simulink model "attitude_controller"  (R2024b)
settings: Solver=ode1  StartTime=0.0  StopTime=120  FixedStep=0.1  RelTol=1e-3
values from neighbouring files (symbols this model uses):
  g0 = 9.81    [main.m]
  m_0 = 6492 * 1000    (= 6492000)    [main.m]
  m_dot_e = T_e_with_losses/v_ex    (= 799.471894568)    [main.m]
  m_p_0 = 4165 * 1000    (= 4165000)    [main.m]
  n_eg_g = 3 + 12    (= 15)    [main.m]
  n_eg_ng = 26    [main.m]
  T_g_full_throttle = T_e_with_losses * n_eg_g    (= 41174801.25)    [main.m]
  T_ng_full_throttle = T_e_with_losses * n_eg_ng    (= 71369655.5)    [main.m]
  theta_0 = deg2rad(90)    [main.m]
  theta_ref = a0 + a1 * t + a2 * t.^2 + a3 * t.^3    [main.m]
libraries: simulink_extras x3, slpidlib x1
settings Model: Creator=jonathanvanzyl  LastModifiedBy=jonathanvanzyl

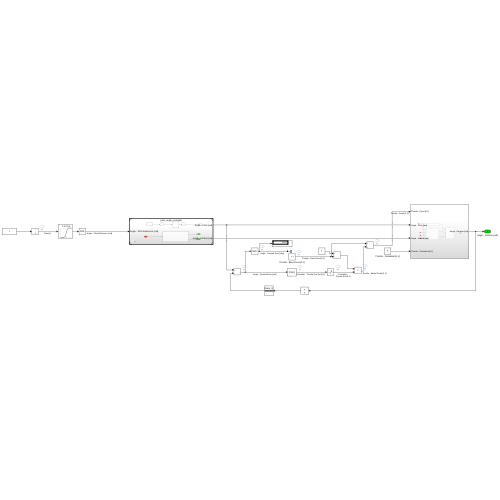
[thumbnail: Simulink's stored preview of the top-level diagram]
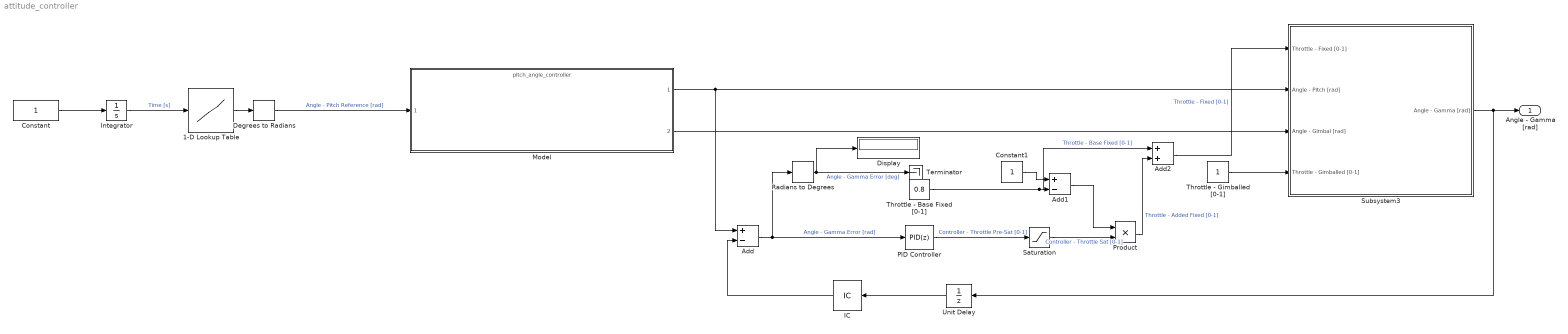
== system attitude_controller ==
  1-D Lookup Table : Lookup_n-D  NumberOfTableDimensions=1  BreakpointsForDimension1=t  Table=theta_ref  InternalRulePriority=Speed  RndMeth=Simplest
  Add : Sum  Inputs=+-
  Add1 : Sum  Inputs=+-
  Add2 : Sum
  Constant : Constant
  Constant1 : Constant
  Degrees to Radians : simulink_extras/Transformations/Degrees to Radians
  Display : Display
  IC : InitialCondition  Value=theta_0
  Integrator : Integrator
  Model : ModelReference  ModelNameDialog=pitch_angle_controller  SimulationMode=Normal  ModelReferenceVersion=1.17
  PID Controller : slpidlib/PID Controller  Controller=PID  Form=Parallel  TimeDomain=Discrete-time  UseExternalTs=off  SampleTime=-1  IntegratorMethod=Forward Euler  FilterMethod=Forward Euler  ControllerParametersSource=internal  P=100  I=0  UseKiTs=off  D=0  UseExternalDerivativeSource=off  N=0.0005  UseFilter=on  TunerSelectOption=Transfer Function Based (PID Tuner App)  InitialConditionSource=internal  InitialConditionForIntegrator=0  InitialConditionForFilter=0  DifferentiatorICPrevScaledInput=0  ExternalReset=none  TrackingMode=off  Kt=1  LimitOutput=off  SatLimitsSource=internal  UpperSaturationLimit=inf  LowerSaturationLimit=-inf  LinearizeAsGain=on  AntiWindupMode=none  Kb=1  LimitIntegrator=off  UpperIntegratorSaturationLimit=inf  LowerIntegratorSaturationLimit=-inf  POutMin=[]  POutMax=[]  IOutMin=[]  IOutMax=[]  DOutMin=[]  DOutMax=[]  NOutMin=[]  NOutMax=[]  SumOutMin=[]  SumOutMax=[]  SaturationOutMin=[]  SaturationOutMax=[]  PParamMin=[]  PParamMax=[]  IParamMin=[]  IParamMax=[]  DParamMin=[]  DParamMax=[]  NParamMin=[]  NParamMax=[]  KbParamMin=[]  KbParamMax=[]  KtParamMin=[]  KtParamMax=[]  KbOutMin=[]  KbOutMax=[]  KtOutMin=[]  KtOutMax=[]  IntegratorOutMin=[]  IntegratorOutMax=[]  FilterOutMin=[]  FilterOutMax=[]  SumI1OutMin=[]  SumI1OutMax=[]  SumI2OutMin=[]  SumI2OutMax=[]  SumI3OutMin=[]  SumI3OutMax=[]  SumI4OutMin=[]  SumI4OutMax=[]  SumDOutMin=[]  SumDOutMax=[]  DifferentiatorOutMin=[]  DifferentiatorOutMax=[]  FilterDiffOutCoefMin=[]  FilterDiffOutCoefMax=[]  ReciprocalOutMin=[]  ReciprocalOutMax=[]  SumDenOutMin=[]  SumDenOutMax=[]  SumNumOutMin=[]  SumNumOutMax=[]  DivideOutMin=[]  DivideOutMax=[]  UdiffTsProdOutMin=[]  UdiffTsProdOutMax=[]  NTsProdOutMin=[]  NTsProdOutMax=[]  UintegralTsProdOutMin=[]  UintegralTsProdOutMax=[]  UngainTsProdOutMin=[]  UngainTsProdOutMax=[]  ClampingZeroOutDataTypeStr=Inherit: Inherit via back propagation  ClampingZeroOutMin=[]  ClampingZeroOutMax=[]  FilterDenConstantOutDataTypeStr=Inherit: Inherit via back propagation  FilterDenConstantOutMin=[]  FilterDenConstantOutMax=[]  PCopyOutDataTypeStr=Inherit: Inherit via back propagation  PCopyOutMin=[]  PCopyOutMax=[]  NCopyOutDataTypeStr=Inherit: Inherit via back propagation  NCopyOutMin=[]  NCopyOutMax=[]  IntegratorContinuousStateAttributes=''  IntegratorStateMustResolveToSignalObject=off  IntegratorRTWStateStorageClass=Auto  FilterContinuousStateAttributes=''  FilterStateMustResolveToSignalObject=off  FilterRTWStateStorageClass=Auto  ParallelPVariant=InternalParameters  IdealPVariant=Disabled  IVariant=InternalParameters  DVariant=InternalParameters  IntegratorVariant=Discrete  SatVariant=Disabled  AWVariant=Passthrough  PCopyVariant=Disabled  TRVariant=Disabled  FdbkBlocksVariant=Forward  IdealPFdbkVariant=Disabled  SatFdbkVariant=Disabled  DerivativeFilterVariant=ForwardEulerFilter  NVariant=InternalParameters  NCopyVariant=Disabled  FilterICVariant=InternalICsFilter  IntegratorICVariant=InternalICs  ExternalResetVariant=Disabled  TRSumVariant=Passthrough  SumFdbkVariant=Disabled  SumVariant=Sum_PID  TsampFilterVariant=InternalTs  TsampNgainVariant=Passthrough  TsampIntegralVariant=Disabled_SignalSpec  ExternalSaturationOutDataTypeStr=Inherit: Same as second input  DerivativeSourceVariant=ErrorSignal  PreIntVariant=InternalPreInt
  Product : Product
  Radians to Degrees : simulink_extras/Transformations/Radians to Degrees
  Saturation : Saturate  UpperLimit=1  LowerLimit=0
  Subsystem3 : Subsystem
  Terminator : Terminator
  Throttle - Base Fixed [0-1] : Constant  Value=0.8
  Throttle - Gimballed [0-1] : Constant
  Unit Delay : UnitDelay  SampleTime=-1  HasFrameUpgradeWarning=on
  Angle - Gamma [rad] : Outport
  wires:
  Model/1 -> Add/1, Subsystem3/2(Angle - Pitch [rad])
  Model/2 -> Subsystem3/3(Angle - Gimbal [rad])
  Throttle - Gimballed [0-1]/1 -> Subsystem3/4(Throttle - Gimballed [0-1])
  Subsystem3/1(Angle - Gamma [rad]) -> Unit Delay/1, Angle - Gamma [rad]/1
  Unit Delay/1 -> IC/1
  IC/1 -> Add/2
  Add/1 -> Radians to Degrees/1, PID Controller/1  "Angle - Gamma Error [rad]"
  Add2/1 -> Subsystem3/1(Throttle - Fixed [0-1])  "Throttle - Fixed [0-1]"
  Constant/1 -> Integrator/1
  Integrator/1 -> 1-D Lookup Table/1  "Time [s]"
  1-D Lookup Table/1 -> Degrees to Radians/1
  Degrees to Radians/1 -> Model/1  "Angle - Pitch Reference [rad]"
  Radians to Degrees/1 -> Display/1, Terminator/1  "Angle - Gamma Error [deg]"
  PID Controller/1 -> Saturation/1  "Controller - Throttle Pre-Sat [0-1]"
  Add1/1 -> Product/1
  Throttle - Base Fixed [0-1]/1 -> Add2/1, Add1/2  "Throttle - Base Fixed [0-1]"
  Constant1/1 -> Add1/1
  Saturation/1 -> Product/2  "Controller - Throttle Sat [0-1]"
  Product/1 -> Add2/2  "Throttle - Added Fixed [0-1]"

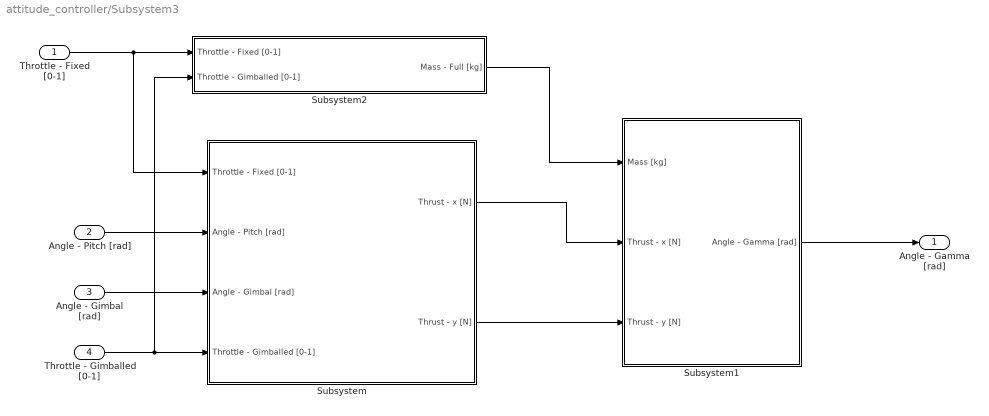
== system attitude_controller/Subsystem3 ==
  Throttle - Fixed [0-1] : Inport
  Angle - Pitch [rad] : Inport  Port=2
  Angle - Gimbal [rad] : Inport  Port=3
  Throttle - Gimballed [0-1] : Inport  Port=4
  Subsystem : Subsystem
  Subsystem1 : Subsystem
  Subsystem2 : Subsystem
  Angle - Gamma [rad] : Outport
  wires:
  Angle - Gimbal [rad]/1 -> Subsystem/3(Angle - Gimbal [rad])
  Subsystem2/1(Mass - Full [kg]) -> Subsystem1/1(Mass [kg])
  Subsystem/1(Thrust - x [N]) -> Subsystem1/2(Thrust - x [N])
  Subsystem/2(Thrust - y [N]) -> Subsystem1/3(Thrust - y [N])
  Angle - Pitch [rad]/1 -> Subsystem/2(Angle - Pitch [rad])
  Throttle - Fixed [0-1]/1 -> Subsystem/1(Throttle - Fixed [0-1]), Subsystem2/1(Throttle - Fixed [0-1])
  Subsystem1/1(Angle - Gamma [rad]) -> Angle - Gamma [rad]/1
  Throttle - Gimballed [0-1]/1 -> Subsystem2/2(Throttle - Gimballed [0-1]), Subsystem/4(Throttle - Gimballed [0-1])

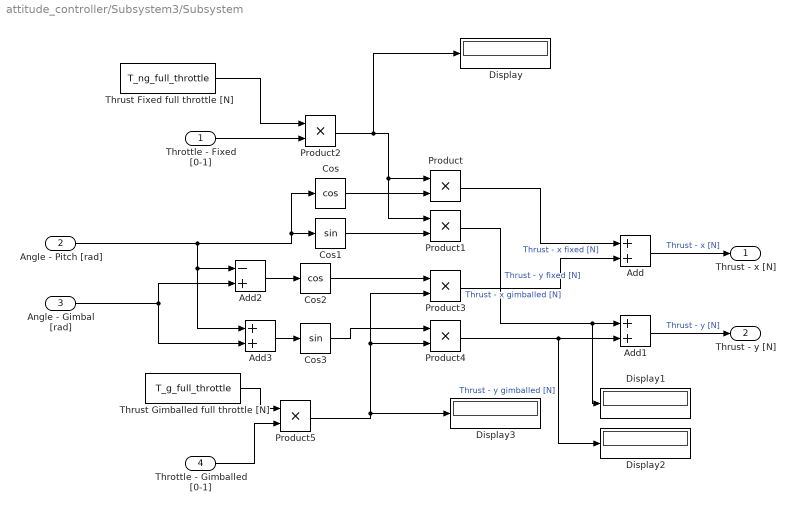
== system attitude_controller/Subsystem3/Subsystem ==
  Throttle - Fixed [0-1] : Inport
  Angle - Pitch [rad] : Inport  Port=2
  Angle - Gimbal [rad] : Inport  Port=3
  Throttle - Gimballed [0-1] : Inport  Port=4
  Add : Sum
  Add1 : Sum
  Add2 : Sum  Inputs=-+
  Add3 : Sum
  Cos : Trigonometry  Operator=cos
  Cos1 : Trigonometry
  Cos2 : Trigonometry  Operator=cos
  Cos3 : Trigonometry
  Display{,1..3} (4 alike) : Display
  Product{,1..5} (6 alike) : Product
  Thrust Fixed full throttle [N] : Constant  Value=T_ng_full_throttle
  Thrust Gimballed full throttle [N] : Constant  Value=T_g_full_throttle
  Thrust - x [N] : Outport
  Thrust - y [N] : Outport  Port=2
  wires:
  Add/1 -> Thrust - x [N]/1  "Thrust - x [N]"
  Thrust Gimballed full throttle [N]/1 -> Product5/1
  Product3/1 -> Add/2  "Thrust - x gimballed [N]"
  Product4/1 -> Display2/1, Add1/2  "Thrust - y gimballed [N]"
  Product5/1 -> Product3/2, Product4/2, Display3/1
  Cos2/1 -> Product3/1
  Angle - Gimbal [rad]/1 -> Add2/2, Add3/2
  Add3/1 -> Cos3/1
  Product/1 -> Add/1  "Thrust - x fixed [N]"
  Throttle - Fixed [0-1]/1 -> Product2/2
  Throttle - Gimballed [0-1]/1 -> Product5/2
  Thrust Fixed full throttle [N]/1 -> Product2/1
  Add2/1 -> Cos2/1
  Cos3/1 -> Product4/1
  Cos/1 -> Product/2
  Angle - Pitch [rad]/1 -> Add3/1, Add2/1, Cos/1, Cos1/1
  Add1/1 -> Thrust - y [N]/1  "Thrust - y [N]"
  Product1/1 -> Display1/1, Add1/1  "Thrust - y fixed [N]"
  Cos1/1 -> Product1/2
  Product2/1 -> Display/1, Product1/1, Product/1

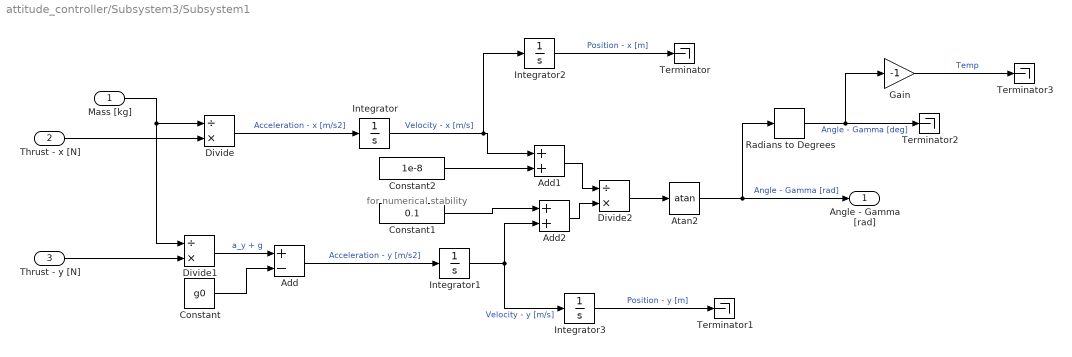
== system attitude_controller/Subsystem3/Subsystem1 ==
  note: for numerical stability
  Mass [kg] : Inport
  Thrust - x [N] : Inport  Port=2
  Thrust - y [N] : Inport  Port=3
  Add : Sum  Inputs=+-
  Add1 : Sum
  Add2 : Sum
  Atan2 : Trigonometry  Operator=atan
  Constant : Constant  Value=g0
  Constant1 : Constant  Value=0.1
  Constant2 : Constant  Value=1e-8
  Divide : Product  Inputs=/*
  Divide1 : Product  Inputs=/*
  Divide2 : Product  Inputs=/*
  Gain : Gain  Gain=-1
  Integrator{,1..3} (4 alike) : Integrator
  Radians to Degrees : simulink_extras/Transformations/Radians to Degrees
  Terminator{,1..3} (4 alike) : Terminator
  Angle - Gamma [rad] : Outport
  wires:
  Divide/1 -> Integrator/1  "Acceleration - x [m/s2]"
  Integrator2/1 -> Terminator/1  "Position - x [m]"
  Add/1 -> Integrator1/1  "Acceleration - y [m/s2]"
  Thrust - x [N]/1 -> Divide/2
  Constant1/1 -> Add2/1
  Integrator/1 -> Integrator2/1, Add1/1  "Velocity - x [m/s]"
  Add2/1 -> Divide2/2
  Integrator1/1 -> Integrator3/1, Add2/2  "Velocity - y [m/s]"
  Atan2/1 -> Radians to Degrees/1, Angle - Gamma [rad]/1  "Angle - Gamma [rad]"
  Thrust - y [N]/1 -> Divide1/2
  Divide1/1 -> Add/1  "a_y + g"
  Divide2/1 -> Atan2/1
  Constant2/1 -> Add1/2
  Add1/1 -> Divide2/1
  Constant/1 -> Add/2
  Integrator3/1 -> Terminator1/1  "Position - y [m]"
  Mass [kg]/1 -> Divide1/1, Divide/1
  Radians to Degrees/1 -> Gain/1, Terminator2/1  "Angle - Gamma [deg]"
  Gain/1 -> Terminator3/1  "Temp"

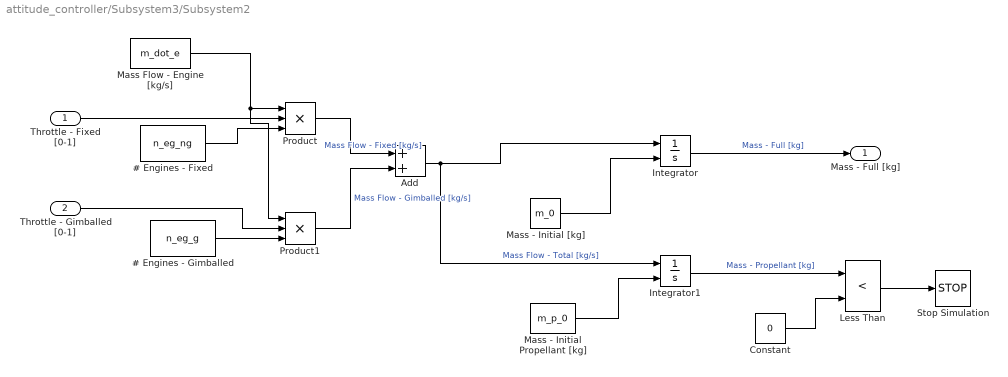
== system attitude_controller/Subsystem3/Subsystem2 ==
  Throttle - Fixed [0-1] : Inport
  Throttle - Gimballed [0-1] : Inport  Port=2
  # Engines - Fixed : Constant  Value=n_eg_ng
  # Engines - Gimballed : Constant  Value=n_eg_g
  Add : Sum
  Constant : Constant  Value=0
  Integrator : Integrator  InitialConditionSource=external
  Integrator1 : Integrator  InitialConditionSource=external
  Less Than : RelationalOperator  Operator=<  OutDataTypeStr=boolean  RndMeth=Simplest  InputSameDT=off
  Mass - Initial Propellant [kg] : Constant  Value=m_p_0
  Mass - Initial [kg] : Constant  Value=m_0
  Mass Flow - Engine [kg/s] : Constant  Value=m_dot_e
  Product : Product  Inputs=3
  Product1 : Product  Inputs=3
  Stop Simulation : Stop
  Mass - Full [kg] : Outport
  wires:
  Throttle - Gimballed [0-1]/1 -> Product1/2
  # Engines - Gimballed/1 -> Product1/3
  Throttle - Fixed [0-1]/1 -> Product/2
  Product1/1 -> Add/2  "Mass Flow - Gimballed [kg/s]"
  Mass - Initial Propellant [kg]/1 -> Integrator1/2
  Mass Flow - Engine [kg/s]/1 -> Product1/1, Product/1
  # Engines - Fixed/1 -> Product/3
  Integrator/1 -> Mass - Full [kg]/1  "Mass - Full [kg]"
  Less Than/1 -> Stop Simulation/1
  Product/1 -> Add/1  "Mass Flow - Fixed [kg/s]"
  Add/1 -> Integrator1/1, Integrator/1  "Mass Flow - Total [kg/s]"
  Integrator1/1 -> Less Than/1  "Mass - Propellant [kg]"
  Mass - Initial [kg]/1 -> Integrator/2
  Constant/1 -> Less Than/2
